simulink model "tri6"  (R2016b)
settings: Solver=VariableStepAuto  StartTime=0.0  StopTime=5  RelTol=1e-3
settings Model: Creator=Admin  LastModifiedBy=Admin

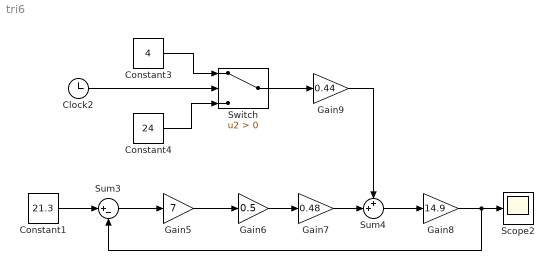
== system tri6 ==
  Clock2 : Clock
  Constant1 : Constant  Value=21.3
  Constant3 : Constant  Value=4
  Constant4 : Constant  Value=24
  Gain5 : Gain  Gain=7
  Gain6 : Gain  Gain=0.5
  Gain7 : Gain  Gain=0.48
  Gain8 : Gain  Gain=14.9
  Gain9 : Gain  Gain=0.44
  Scope2 : Scope
  Sum3 : Sum  Inputs=|+-
  Sum4 : Sum  Inputs=++|
  Switch : Switch  Criteria=u2 > Threshold
  wires:
  Gain6/1 -> Gain7/1
  Constant1/1 -> Sum3/1
  Sum3/1 -> Gain5/1
  Gain5/1 -> Gain6/1
  Gain7/1 -> Sum4/2
  Sum4/1 -> Gain8/1
  Gain8/1 -> Sum3/2, Scope2/1
  Gain9/1 -> Sum4/1
  Switch/1 -> Gain9/1
  Clock2/1 -> Switch/2
  Constant3/1 -> Switch/1
  Constant4/1 -> Switch/3
